simulink model "Smart_Solar_Water_Heating_G1"  (R2024a)
settings: Solver=ode45  StartTime=0.0  StopTime=86400  MaxStep=60  RelTol=1e-3
model workspace (MAT data in the model file):
  Cp = 4186
  ON_OFF_switch = 1
  T_cold = 25
  T_setpoint = 40
  T_solar_max = 70
  flow_rate = 0.01
settings Model: Creator=User  LastModifiedBy=User

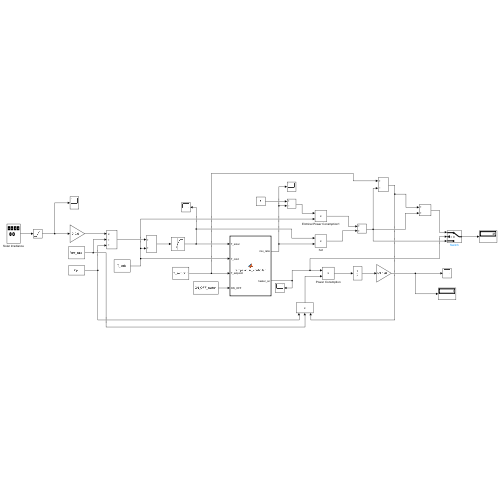
[thumbnail: Simulink's stored preview of the top-level diagram]
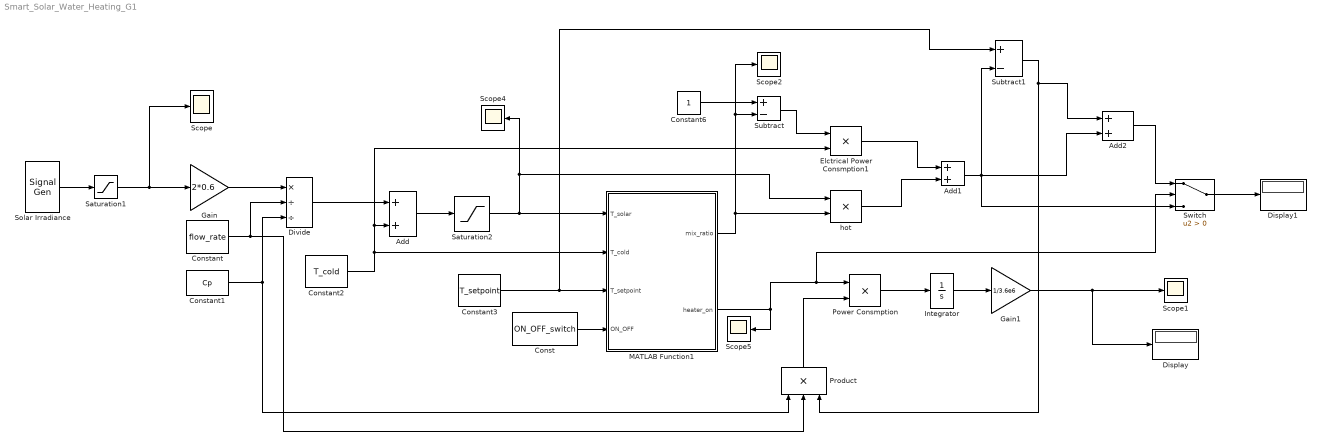
== system Smart_Solar_Water_Heating_G1 ==
  Add : Sum
  Add1 : Sum
  Add2 : Sum
  Const : Constant  Value=ON_OFF_switch  SampleTime=-1
  Constant : Constant  Value=flow_rate  SampleTime=-1
  Constant1 : Constant  Value=Cp  SampleTime=-1
  Constant2 : Constant  Value=T_cold  SampleTime=-1
  Constant3 : Constant  Value=T_setpoint  SampleTime=-1
  Constant6 : Constant  SampleTime=-1
  Display : Display
  Display1 : Display
  Divide : Product  Inputs=*//
  Elctrical Power Consmption1 : Product
  Gain : Gain  Gain=2*0.6
  Gain1 : Gain  Gain=1/3.6e6
  Integrator : Integrator
  MATLAB Function1 : MATLAB Function  TreatAsAtomicUnit=on
  Power Consmption : Product
  Product : Product  Inputs=3
  Saturation1 : Saturate  UpperLimit=1000  LowerLimit=0
  Saturation2 : Saturate  UpperLimit=T_solar_max  LowerLimit=T_cold
  Scope{,1..2,4..5} (5 alike) : Scope
  Solar Irradiance : SignalGenerator  Amplitude=900  Frequency=1/(24*3600)
  Subtract : Sum  Inputs=+-
  Subtract1 : Sum  Inputs=+-
  Switch : Switch  Criteria=u2 > Threshold  SaturateOnIntegerOverflow=off  InputSameDT=off
  hot : Product
  wires:
  Solar Irradiance/1 -> Saturation1/1
  Gain/1 -> Divide/1
  Saturation1/1 -> Scope/1, Gain/1
  Constant/1 -> Product/2, Divide/2
  Constant1/1 -> Product/1, Divide/3
  Divide/1 -> Add/1
  Constant2/1 -> MATLAB Function1/2(T_cold), Add/2, Elctrical Power Consmption1/2
  Add/1 -> Saturation2/1
  Saturation2/1 -> hot/1, Scope4/1, MATLAB Function1/1(T_solar)
  Constant3/1 -> Subtract1/1, MATLAB Function1/3(T_setpoint)
  MATLAB Function1/2(heater_on) -> Switch/2, Power Consmption/1, Scope5/1
  Power Consmption/1 -> Integrator/1
  Integrator/1 -> Gain1/1
  MATLAB Function1/1(mix_ratio) -> Scope2/1, Subtract/2, hot/2
  Constant6/1 -> Subtract/1
  Subtract/1 -> Elctrical Power Consmption1/1
  Elctrical Power Consmption1/1 -> Add1/1
  hot/1 -> Add1/2
  Add1/1 -> Subtract1/2, Add2/2, Switch/3
  Switch/1 -> Display1/1
  Gain1/1 -> Display/1, Scope1/1
  Subtract1/1 -> Product/3, Add2/1
  Product/1 -> Power Consmption/2
  Add2/1 -> Switch/1
  Const/1 -> MATLAB Function1/4(ON_OFF)

== matlab function Smart_Solar_Water_Heating_G1/MATLAB Function1 ==
  data: T_solar input; mix_ratio output; T_cold input; T_setpoint input; heater_on output; ON_OFF input
function [mix_ratio, heater_on] = temperature_controller(T_solar, T_cold, T_setpoint , ON_OFF)
       
    if T_solar >= T_setpoint
        % Solar water is too hot
        % Mix with cold water, turn heater OFF
        heater_on = 0;
        
        if T_solar > T_cold
            mix_ratio = (T_setpoint - T_cold) / (T_solar - T_cold);
        else
            mix_ratio = 1;
        end
        
        % Clamp mix_ratio between 0 and 1
        mix_ratio = max(0, min(1, mix_ratio));
                
    else
        % Solar water is too cold
        % No mixing, turn heater ON
        
        mix_ratio = 1;  % Use 100% solar water
        if ON_OFF == 1 % hot water shower status
            heater_on = 1;
        else
            heater_on = 0;
        end
    end
end
